simulink model "CILab11Noisy"  (R2016b)
settings: Solver=VariableStepAuto  StartTime=0.0  StopTime=10.0  RelTol=1e-3
libraries: simulink x1, fuzblock x1
settings Model: Creator=user  LastModifiedBy=user

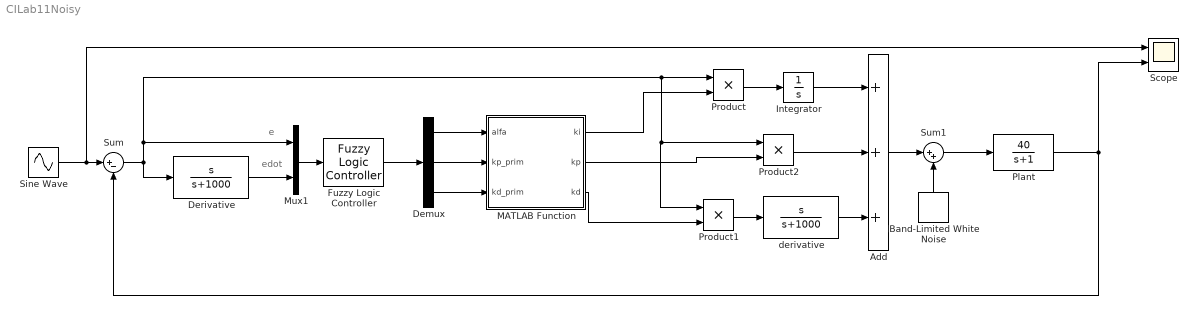
== system CILab11Noisy ==
  note: edot
  note: e
  Add : Sum  Inputs=+++
  Band-Limited White Noise : simulink/Sources/Band-Limited White Noise  Cov=[0.001]  Ts=0.1  seed=[23341]
  Demux : Demux  Outputs=3
  Derivative : TransferFcn  Numerator=[1,0]  Denominator=[1 1000]
  Fuzzy Logic Controller : fuzblock/Fuzzy Logic  Controller  fis=['Untitled.fis']
  Integrator : Integrator
  MATLAB Function : MATLAB Function  TreatAsAtomicUnit=on
  Mux1 : Mux  Inputs=2
  Plant : TransferFcn  Numerator=[40]  Denominator=[1 1]
  Product : Product
  Product1 : Product
  Product2 : Product
  Scope : Scope  NumInputPorts=2
  Sine Wave : Sin  SampleTime=0
  Sum : Sum  Inputs=|+-
  Sum1 : Sum  Inputs=|++
  derivative : TransferFcn  Numerator=[1,0]  Denominator=[1 1000]
  wires:
  Fuzzy Logic Controller/1 -> Demux/1
  Demux/1 -> MATLAB Function/1(alfa)
  Demux/2 -> MATLAB Function/2(kp_prim)
  Demux/3 -> MATLAB Function/3(kd_prim)
  Sine Wave/1 -> Scope/1, Sum/1
  Sum/1 -> Derivative/1, Mux1/1, Product1/1, Product2/1, Product/1
  Mux1/1 -> Fuzzy Logic Controller/1
  Integrator/1 -> Add/1
  derivative/1 -> Add/3
  MATLAB Function/1(ki) -> Product/2
  Product/1 -> Integrator/1
  Product2/1 -> Add/2
  MATLAB Function/2(kp) -> Product2/2
  Product1/1 -> derivative/1
  MATLAB Function/3(kd) -> Product1/2
  Derivative/1 -> Mux1/2
  Band-Limited White Noise/1 -> Sum1/2
  Plant/1 -> Scope/2, Sum/2
  Add/1 -> Sum1/1
  Sum1/1 -> Plant/1

== matlab function CILab11Noisy/MATLAB Function ==
  data: alfa input; ki output; kp_prim input; kd_prim input; kp output; kd output
function [ki,kp,kd] = fcn(alfa,kp_prim,kd_prim)
kp = 5*kp_prim;
kd = 5*kd_prim;
ki = (kp^2)/(alfa*kd);

% ki=kd/a;
